simulink model "CDMA2000sint_C_etapa1"  (R2012b)
settings: Solver=ode45  StartTime=0.0  StopTime=10.0  RelTol=1e-3
libraries: commcnvcod2 x2, commrandsrc2 x1
settings Model: Creator=student  LastModifiedBy=student

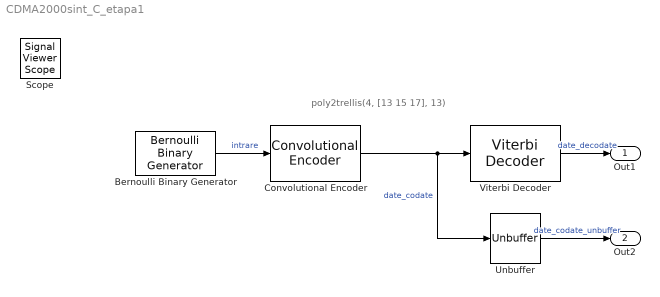
== system CDMA2000sint_C_etapa1 ==
  note: poly2trellis(4, [13 15 17], 13)
  Bernoulli Binary Generator : commrandsrc2/Bernoulli Binary Generator  P=0.5  seed=61  Ts=1  frameBased=off  sampPerFrame=1  orient=off  outDataType=double
  Convolutional Encoder : commcnvcod2/Convolutional Encoder  trellis=poly2trellis(4, [13 15 17], 13)  opMode=Continuous  DelayedResetAction=off  hasIniStPort=off  hasFinStPort=off  usePuncVector=off  punctureVector=[1; 1; 0; 1; 0; 1]  reset=Unused parameter value
  Unbuffer : Unbuffer  SampleBasedProcessing=Same as frame based
  Viterbi Decoder : commcnvcod2/Viterbi Decoder  trellis=poly2trellis(4, [13 15 17], 13)  isPunctured=off  punctureVector=[1; 1; 0; 1; 0; 1]  erasures=off  dectype=Hard decision  runSigValErrCheck=off  nsdecb=4  smWordLength=16  tbdepth=1  opmode=Continuous  reset=off  outDataType=Inherit via internal rule  delayedResetAction=off
  Out1 : Outport
  Out2 : Outport  Port=2
  Scope : SignalViewerScope  IOType=viewer  NumInputPorts=3  RefreshTime=0.035000
      settings: ShowDataMarkers=on  YMin=-5~-5~-5  YMax=5~5~5
  wires:
  Bernoulli Binary Generator/1 -> Convolutional Encoder/1  "intrare"
  Convolutional Encoder/1 -> Unbuffer/1, Viterbi Decoder/1  "date_codate"
  Viterbi Decoder/1 -> Out1/1  "date_decodate"
  Unbuffer/1 -> Out2/1  "date_codate_unbuffer"
